simulink model "GlucagonGlucoseIntegration"  (R2019a)
settings: Solver=VariableStepAuto  StartTime=0.0  StopTime=500  RelTol=1e-3
undefined symbols (not defined in the file): GAMMA_B, GHC_B, GLC_B, GPT_B, IHC_B, IPT_B, Q_i_P, r_bHGP, r_bHGU, V_i_PF
settings Model: Creator=rache  LastModifiedBy=rache

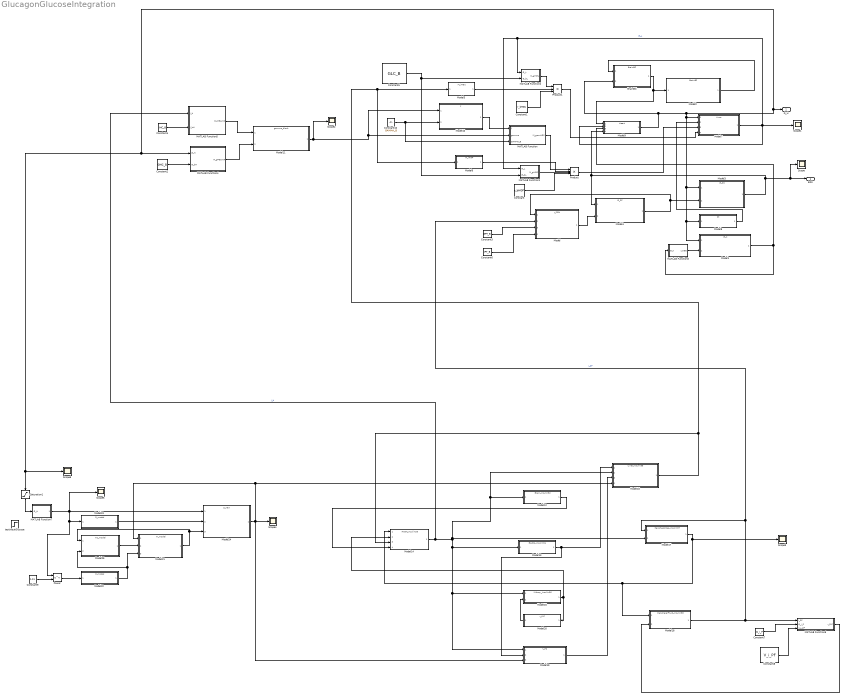
== system GlucagonGlucoseIntegration ==
  BrainBC : ModelReference  ModelNameDialog=BrainBC  SimulationMode=Normal  ModelReferenceVersion=1.6
  Constant : Constant  Value=r_bHGP
  Constant1 : Constant  Value=r_bHGU
  Constant10 : Constant  Value=GAMMA_B
  Constant2 : Constant  Value=GHC_B
  Constant3 : Constant  Value=GPT_B
  Constant4 : Constant  Value=IHC_B
  Constant5 : Constant  Value=GLC_B
  Constant6 : Constant  Value=IPT_B
  Constant7 : Constant  Value=Q_i_P
  Constant8 : Constant  Value=V_i_PF
  Constant9 : Constant  Value=1.11
  MATLAB Function : MATLAB Function  TreatAsAtomicUnit=on
  MATLAB Function1 : MATLAB Function  TreatAsAtomicUnit=on
  MATLAB Function2 : MATLAB Function  TreatAsAtomicUnit=on
  MATLAB Function3 : MATLAB Function  TreatAsAtomicUnit=on
  MATLAB Function4 : MATLAB Function  TreatAsAtomicUnit=on
  MATLAB Function5 : MATLAB Function  TreatAsAtomicUnit=on
  MATLAB Function6 : MATLAB Function  TreatAsAtomicUnit=on
  MATLAB Function7 : MATLAB Function  TreatAsAtomicUnit=on
  Model : ModelReference  ModelNameDialog=r_PGU  SimulationMode=Normal  ModelReferenceVersion=1.5
  Model1 : ModelReference  ModelNameDialog=G_K  SimulationMode=Normal  ModelReferenceVersion=1.4
  Model10 : ModelReference  ModelNameDialog=f  SimulationMode=Normal  ModelReferenceVersion=1.10
  Model11 : ModelReference  ModelNameDialog=gamma_block  SimulationMode=Normal  ModelReferenceVersion=1.5
  Model12 : ModelReference  ModelNameDialog=Brain_Insulin32  SimulationMode=Normal  ModelReferenceVersion=1.3
  Model13 : ModelReference  ModelNameDialog=Gastro_Insulin34  SimulationMode=Normal  ModelReferenceVersion=1.3
  Model14 : ModelReference  ModelNameDialog=Heart_Insulin33  SimulationMode=Normal  ModelReferenceVersion=1.6
  Model15 : ModelReference  ModelNameDialog=Kidney_Insulin36  SimulationMode=Normal  ModelReferenceVersion=1.7
  Model16 : ModelReference  ModelNameDialog=Liver_Insulin35  SimulationMode=Normal  ModelReferenceVersion=1.7
  Model17 : ModelReference  ModelNameDialog=PeripheralCap_Insulin37  SimulationMode=Normal  ModelReferenceVersion=1.5
  Model18 : ModelReference  ModelNameDialog=PeripheralFluid_Insulin38  SimulationMode=Normal  ModelReferenceVersion=1.4
  Model19 : ModelReference  ModelNameDialog=r_LIC  SimulationMode=Normal  ModelReferenceVersion=1.2
  Model2 : ModelReference  ModelNameDialog=BrainBF  SimulationMode=Normal  ModelReferenceVersion=1.6
  Model20 : ModelReference  ModelNameDialog=r_KIC  SimulationMode=Normal  ModelReferenceVersion=1.1
  Model21 : ModelReference  ModelNameDialog=m_model  SimulationMode=Normal  ModelReferenceVersion=1.2
  Model22 : ModelReference  ModelNameDialog=P_model  SimulationMode=Normal  ModelReferenceVersion=1.9
  Model23 : ModelReference  ModelNameDialog=R_model.slx  SimulationMode=Normal  ModelReferenceVersion=1.8
  Model24 : ModelReference  ModelNameDialog=S_new  SimulationMode=Normal  ModelReferenceVersion=1.4
  Model25 : ModelReference  ModelNameDialog=ms_model  SimulationMode=Normal  ModelReferenceVersion=1.3
  Model3 : ModelReference  ModelNameDialog=G_PC  SimulationMode=Normal  ModelReferenceVersion=1.5
  Model4 : ModelReference  ModelNameDialog=G_PF  SimulationMode=Normal  ModelReferenceVersion=1.3
  Model5 : ModelReference  ModelNameDialog=M_iHGU  SimulationMode=Normal  ModelReferenceVersion=1.4
  Model6 : ModelReference  ModelNameDialog=M_iHGP  SimulationMode=Normal  ModelReferenceVersion=1.2
  Model7 : ModelReference  ModelNameDialog=Liver  SimulationMode=Normal  ModelReferenceVersion=1.6
  Model8 : ModelReference  ModelNameDialog=GI  SimulationMode=Normal  ModelReferenceVersion=1.4
  Model9 : ModelReference  ModelNameDialog=Heart  SimulationMode=Normal  ModelReferenceVersion=1.4
  Power : Math  Operator=pow  SaturateOnIntegerOverflow=on
  Product : Product  Inputs=4
  Product1 : Product  Inputs=3
  Saturation1 : Saturate  UpperLimit=inf  LowerLimit=0
  Scope{,1..6} (7 alike) : Scope
  testInputGlucose : Step  Before=160  After=200  SampleTime=0
  BGV : Outport  OutMin=0
  G_H : Outport  Port=2  OutMin=0
  wires:
  Model7/1 -> MATLAB Function2/1(G_L), MATLAB Function1/1(G_L), Scope1/1, Model9/2  "G_L"
  Model1/1 -> Model9/3, MATLAB Function3/1(G_K)
  Model4/1 -> Model/1, Model3/2
  Product/1 -> Model7/3
  Product1/1 -> Model7/4
  Model/1 -> Model4/2
  Constant3/1 -> Model/3
  Model11/1 -> Scope2/1, Model10/1, MATLAB Function/2(gamma)
  MATLAB Function/1(M_gamHGP) -> Product/1
  MATLAB Function3/1(r_KGE) -> Model1/2
  Constant5/1 -> MATLAB Function1/2(G_bL), MATLAB Function2/2(G_bL)
  Constant6/1 -> Model/4
  Constant1/1 -> Product1/3
  Model5/1 -> Product1/2
  Constant/1 -> Product/4
  BrainBC/1 -> Model9/1, Model2/1
  Model16/1 -> Model14/3, Model6/1, Model5/1
  Model6/1 -> Product/2
  MATLAB Function2/1(M_gHGU) -> Product1/1
  Model2/1 -> BrainBC/1
  Model10/1 -> MATLAB Function/1(f)
  Model8/1 -> Model7/2
  MATLAB Function1/1(M_gHGP) -> Product/3
  Model3/1 -> Model4/1, Model9/4, Scope/1, BGV/1
  Constant4/1 -> MATLAB Function5/2(I_bH)
  MATLAB Function4/1(M_gPGamR) -> Model11/2
  MATLAB Function5/1(M_iPGamR) -> Model11/1
  Constant2/1 -> MATLAB Function4/2(G_bH)
  Model13/1 -> Model19/2, Model16/1
  Model18/1 -> Model/2, Model17/1, MATLAB Function6/1(I_PF)  "I_PF"
  Model17/1 -> Scope3/1, Model14/1, Model18/1
  Model19/1 -> Model16/3
  Constant7/1 -> MATLAB Function6/2(Q_i_P)
  Model20/1 -> Model15/2
  Model12/1 -> Model14/4
  MATLAB Function6/1(r_PIC) -> Model18/2
  Model15/1 -> Model14/2, Model20/1
  Constant8/1 -> MATLAB Function6/3(V_i_PF)
  Model14/1 -> MATLAB Function5/1(I_H), Model16/2, Model12/1, Model17/2, Model13/1, Model15/1, Model19/1  "I_H"
  Model9/1 -> Model3/1, Model8/1, Model1/1, Model7/1, MATLAB Function4/1(G_H), Scope6/1, Saturation1/1, G_H/1, BrainBC/2
  Power/1 -> Model22/1
  Constant9/1 -> Power/2
  Model22/1 -> Model25/2, Model21/3
  Model21/1 -> Model25/1, Model24/3
  Model23/1 -> Model24/2
  Model24/1 -> Model16/4, Model21/1, Model19/3, Scope4/1
  Model25/1 -> Model21/2
  MATLAB Function7/1(X) -> Scope5/1, Power/1, Model23/1, Model24/1
  Saturation1/1 -> MATLAB Function7/1(G_H)
  Constant10/1 -> MATLAB Function/3(GAMMA_B), Model10/2

== matlab function GlucagonGlucoseIntegration/MATLAB Function1 ==
  data: G_L input; M_gHGP output; G_bL input
function M_gHGP = fcn(G_L, G_bL)

M_gHGP = 1.42 - 1.41*tanh(0.62*(G_L/G_bL - 0.497));

== matlab function GlucagonGlucoseIntegration/MATLAB Function ==
  data: f input; M_gamHGP output; gamma input; GAMMA_B input
function M_gamHGP = fcn(f, gamma, GAMMA_B)
M_gamHGP = 2.7*tanh(0.39*gamma/GAMMA_B) - f;

== matlab function GlucagonGlucoseIntegration/MATLAB Function2 ==
  data: G_L input; M_gHGU output; G_bL input
function M_gHGU = fcn(G_L, G_bL)

M_gHGU = 5.66*(1 + tanh(2.44*(G_L/G_bL - 1.48)));

== matlab function GlucagonGlucoseIntegration/MATLAB Function3 ==
  data: G_K input; r_KGE output
function r_KGE = fcn(G_K)

r_KGE = 71+(71*tanh(0.11*(G_K - 460)));

== matlab function GlucagonGlucoseIntegration/MATLAB Function4 ==
  data: G_H input; M_gPGamR output; G_bH input
function M_gPGamR = fcn(G_H, G_bH)
M_gPGamR = 1.31 - 0.61*tanh(1.06*(G_H/G_bH - 0.47));

== matlab function GlucagonGlucoseIntegration/MATLAB Function5 ==
  data: I_H input; M_iPGamR output; I_bH input
function M_iPGamR = fcn(I_H, I_bH)

M_iPGamR = 2.93 - 2.09*(tanh(4.18*(I_H/I_bH - 0.62)));

== matlab function GlucagonGlucoseIntegration/MATLAB Function6 ==
  data: I_PF input; r_PIC output; Q_i_P input; V_i_PF input
function r_PIC = fcn(I_PF, Q_i_P, V_i_PF)
r_PIC=I_PF/(((1-0.15)/(0.15*Q_i_P))-(20/V_i_PF));

== matlab function GlucagonGlucoseIntegration/MATLAB Function7 ==
  data: G_H input; X output
function X = X_function(G_H)
%X_FUNCTION Calculate X from G_H (glucose output of heart)
%   Inputs: G_H (g)
%   Outputs: X (glucose enhanced excitation factor)
num = G_H^3.27;
denom = (132^3.27 + 5.93*((G_H)^3.02));
X = num/denom;
end
